simulink library "halin"  (R2021b)
settings: Solver=VariableStepAuto  StartTime=0.0  StopTime=10.0  RelTol=1e-3
undefined symbols (not defined in the file): TRUE
libraries: FVT_lib x177, hcu_lib x55
(part 12 of 17)

== system halin/HAL_IN/CAN5/VHAL_CANMsgInvalidTBOX1_flg ==
  Cast To Boolean13 : DataTypeConversion  OutDataTypeStr=boolean
  Constant : Constant  Value=TRUE
  Latch13 : hcu_lib/Basic_Blocks/Latch
  Switch13 : Switch  Criteria=u2 ~= 0
  Unit Delay : UnitDelay  SampleTime=-1  HasFrameUpgradeWarning=on
  UnitConverter : DataTypeConversion  OutDataTypeStr=boolean
  Out : Outport
  wires:
  Constant/1 -> Switch13/3
  Unit Delay/1 -> Cast To Boolean13/1
  Cast To Boolean13/1 -> Switch13/1, Latch13/1
  Switch13/1 -> UnitConverter/1
  Latch13/1 -> Switch13/2
  UnitConverter/1 -> Unit Delay/1, Out/1  "VHAL_CANMsgInvalidTBOX1_flg"

== system halin/HAL_IN/CAN5/VHAL_CANMsgInvalidTBOX2_flg ==
  Cast To Boolean13 : DataTypeConversion  OutDataTypeStr=boolean
  Constant : Constant  Value=TRUE
  Latch13 : hcu_lib/Basic_Blocks/Latch
  Switch13 : Switch  Criteria=u2 ~= 0
  Unit Delay : UnitDelay  SampleTime=-1  HasFrameUpgradeWarning=on
  UnitConverter : DataTypeConversion  OutDataTypeStr=boolean
  Out : Outport
  wires:
  Constant/1 -> Switch13/3
  Unit Delay/1 -> Cast To Boolean13/1
  Cast To Boolean13/1 -> Switch13/1, Latch13/1
  Switch13/1 -> UnitConverter/1
  Latch13/1 -> Switch13/2
  UnitConverter/1 -> Unit Delay/1, Out/1  "VHAL_CANMsgInvalidTBOX2_flg"

== system halin/HAL_IN/CAN5/VHAL_CANMsgInvalidTBOX3_flg ==
  Cast To Boolean13 : DataTypeConversion  OutDataTypeStr=boolean
  Constant : Constant  Value=TRUE
  Latch13 : hcu_lib/Basic_Blocks/Latch
  Switch13 : Switch  Criteria=u2 ~= 0
  Unit Delay : UnitDelay  SampleTime=-1  HasFrameUpgradeWarning=on
  UnitConverter : DataTypeConversion  OutDataTypeStr=boolean
  Out : Outport
  wires:
  Constant/1 -> Switch13/3
  Unit Delay/1 -> Cast To Boolean13/1
  Cast To Boolean13/1 -> Switch13/1, Latch13/1
  Switch13/1 -> UnitConverter/1
  Latch13/1 -> Switch13/2
  UnitConverter/1 -> Unit Delay/1, Out/1  "VHAL_CANMsgInvalidTBOX3_flg"

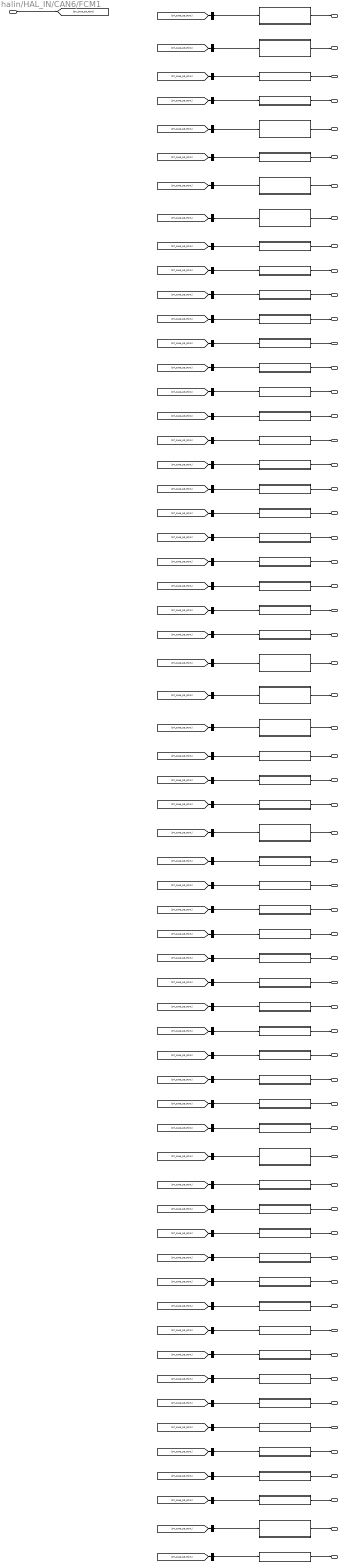
== system halin/HAL_IN/CAN6/FCM1 ==
  DT_CAN6_SG_FCM1 : Inport
  ACCComfortBandLower : Subsystem
  ACCComfortBandUpper : Subsystem
  ACCJerkLowerLimit : Subsystem
  ACCJerkUpperLimit : Subsystem
  ACCObjDist : Subsystem
  ACCObjDstLvl : Subsystem
  ACCObjRelSpd : Subsystem
  ACCRequiredAccel : Subsystem
  ACCTakeoverReq : Subsystem
  ACCVehHoldReq : Subsystem
  ADASACCSta : Subsystem
  ADASAEBReq : Subsystem
  ADASAEBSta : Subsystem
  ADASCAMSpdLim : Subsystem
  ADASDBSReq : Subsystem
  ADASFCWMute : Subsystem
  ADASFCWSta : Subsystem
  ADASFaultSta : Subsystem
  ADASFltWrnReq : Subsystem
  ADASForceIdle : Subsystem
  ADASISASta : Subsystem
  ADASLDWMute : Subsystem
  ADASLDWSta : Subsystem
  ADASLFCHandsOffWarning : Subsystem
  ADASLFCSta : Subsystem
  ADASLFCWarnSound : Subsystem
  ADASLKASta : Subsystem
  ADASLaneModeL : Subsystem
  ADASLaneModeR : Subsystem
  ADASLanecurveL : Subsystem
  ADASLanecurveR : Subsystem
  ADASLanetypeL : Subsystem
  ADASLanetypeR : Subsystem
  ADASSLIFSpdLim : Subsystem
  ADASSLIFSta : Subsystem
  ADASShftPosnReq : Subsystem
  ADASShftPosnReqA : Subsystem
  ADASVehSpdLim : Subsystem
  ADASWarningMsg : Subsystem
  AEBVehHoldReq : Subsystem
  CameraBlockage : Subsystem
  FCM1Checksum : Subsystem
  FCM1LifeCount : Subsystem
  FCMACCmode : Subsystem
  FCMLKAStrToqReq : Subsystem
  FCMLKATOIAct : Subsystem
  FCMLKATOIFault : Subsystem
  ForceLowBeam : Subsystem
  HazardWarningReq : Subsystem
  ISAWarningMsg : Subsystem
  LKAHODDisplayWarning : Subsystem
  LKAHODSoundWarning : Subsystem
  LVDAACCStatusInformation : Subsystem
  LVDADisabled : Subsystem
  LVDAFailinfo : Subsystem
  LVDAMuteSta : Subsystem
  LVDAWarning : Subsystem
  LeftTurnLightReq : Subsystem
  RightTurnLightReq : Subsystem
  TargetType : Subsystem
  TimeGapLevel : Subsystem
  bus_selector : BusSelector  OutputSignals=CAN6_ACC_ComfortBandLower
  bus_selector1 : BusSelector  OutputSignals=CAN6_ACC_ComfortBandUpper
  bus_selector10 : BusSelector  OutputSignals=CAN6_ADAS_ACC_Sta
  bus_selector11 : BusSelector  OutputSignals=CAN6_ADAS_AEBReq
  bus_selector12 : BusSelector  OutputSignals=CAN6_ADAS_AEB_Sta
  bus_selector13 : BusSelector  OutputSignals=CAN6_ADAS_CAM_SpdLim
  bus_selector14 : BusSelector  OutputSignals=CAN6_ADAS_DBSReq
  bus_selector15 : BusSelector  OutputSignals=CAN6_ADAS_FCW_Mute
  bus_selector16 : BusSelector  OutputSignals=CAN6_ADAS_FCW_Sta
  bus_selector17 : BusSelector  OutputSignals=CAN6_ADAS_FaultSta
  bus_selector18 : BusSelector  OutputSignals=CAN6_ADAS_FltWrnReq
  bus_selector19 : BusSelector  OutputSignals=CAN6_ADAS_ForceIdle
  bus_selector2 : BusSelector  OutputSignals=CAN6_ACC_JerkLowerLimit
  bus_selector20 : BusSelector  OutputSignals=CAN6_ADAS_ISA_Sta
  bus_selector21 : BusSelector  OutputSignals=CAN6_ADAS_LDW_Mute
  bus_selector22 : BusSelector  OutputSignals=CAN6_ADAS_LDW_Sta
  bus_selector23 : BusSelector  OutputSignals=CAN6_ADAS_LFC_Hands_Off_Warning
  bus_selector24 : BusSelector  OutputSignals=CAN6_ADAS_LFC_Sta
  bus_selector25 : BusSelector  OutputSignals=CAN6_ADAS_LFC_Warn_Sound
  bus_selector26 : BusSelector  OutputSignals=CAN6_ADAS_LKA_Sta
  bus_selector27 : BusSelector  OutputSignals=CAN6_ADAS_LaneModeL
  bus_selector28 : BusSelector  OutputSignals=CAN6_ADAS_LaneModeR
  bus_selector29 : BusSelector  OutputSignals=CAN6_ADAS_Lane_curveL
  bus_selector3 : BusSelector  OutputSignals=CAN6_ACC_JerkUpperLimit
  bus_selector30 : BusSelector  OutputSignals=CAN6_ADAS_Lane_curveR
  bus_selector31 : BusSelector  OutputSignals=CAN6_ADAS_LanetypeL
  bus_selector32 : BusSelector  OutputSignals=CAN6_ADAS_LanetypeR
  bus_selector33 : BusSelector  OutputSignals=CAN6_ADAS_SLIF_SpdLim
  bus_selector34 : BusSelector  OutputSignals=CAN6_ADAS_SLIF_Sta
  bus_selector35 : BusSelector  OutputSignals=CAN6_ADAS_ShftPosnReq
  bus_selector36 : BusSelector  OutputSignals=CAN6_ADAS_ShftPosnReq_A
  bus_selector37 : BusSelector  OutputSignals=CAN6_ADAS_VehSpdLim
  bus_selector38 : BusSelector  OutputSignals=CAN6_ADAS_WarningMsg
  bus_selector39 : BusSelector  OutputSignals=CAN6_AEB_VehHoldReq
  bus_selector4 : BusSelector  OutputSignals=CAN6_ACC_ObjDist
  bus_selector40 : BusSelector  OutputSignals=CAN6_CameraBlockage
  bus_selector41 : BusSelector  OutputSignals=CAN6_FCM1_Checksum
  bus_selector42 : BusSelector  OutputSignals=CAN6_FCM1_LifeCount
  bus_selector43 : BusSelector  OutputSignals=CAN6_FCM_ACCmode
  bus_selector44 : BusSelector  OutputSignals=CAN6_FCM_LKA_StrToqReq
  bus_selector45 : BusSelector  OutputSignals=CAN6_FCM_LKA_TOIAct
  bus_selector46 : BusSelector  OutputSignals=CAN6_FCM_LKA_TOIFault
  bus_selector47 : BusSelector  OutputSignals=CAN6_ForceLowBeam
  bus_selector48 : BusSelector  OutputSignals=CAN6_HazardWarningReq
  bus_selector49 : BusSelector  OutputSignals=CAN6_ISA_WarningMsg
  bus_selector5 : BusSelector  OutputSignals=CAN6_ACC_ObjDstLvl
  bus_selector50 : BusSelector  OutputSignals=CAN6_LKA_HOD_Display_Warning
  bus_selector51 : BusSelector  OutputSignals=CAN6_LKA_HOD_Sound_Warning
  bus_selector52 : BusSelector  OutputSignals=CAN6_LVDA_ACCStatusInformation
  bus_selector53 : BusSelector  OutputSignals=CAN6_LVDA_Disabled
  bus_selector54 : BusSelector  OutputSignals=CAN6_LVDA_Failinfo
  bus_selector55 : BusSelector  OutputSignals=CAN6_LVDA_Mute_Sta
  bus_selector56 : BusSelector  OutputSignals=CAN6_LVDA_Warning
  bus_selector57 : BusSelector  OutputSignals=CAN6_LeftTurnLightReq
  bus_selector58 : BusSelector  OutputSignals=CAN6_RightTurnLightReq
  bus_selector59 : BusSelector  OutputSignals=CAN6_Target_Type
  bus_selector6 : BusSelector  OutputSignals=CAN6_ACC_ObjRelSpd
  bus_selector60 : BusSelector  OutputSignals=CAN6_TimeGapLevel
  bus_selector7 : BusSelector  OutputSignals=CAN6_ACC_RequiredAccel
  bus_selector8 : BusSelector  OutputSignals=CAN6_ACC_TakeoverReq
  bus_selector9 : BusSelector  OutputSignals=CAN6_ACC_VehHoldReq
  VHAL_ACCComfortBandLower_mps2 : Outport
  VHAL_ACCComfortBandUpper_mps2 : Outport  Port=2
  VHAL_ACCJerkLowerLimit_mps3 : Outport  Port=3
  VHAL_ACCJerkUpperLimit_mps3 : Outport  Port=4
  VHAL_ACCObjDist_m : Outport  Port=5
  VHAL_ACCObjDstLvl_enum : Outport  Port=6
  VHAL_ACCObjRelSpd_mps : Outport  Port=7
  VHAL_ACCRequiredAccel_mps2 : Outport  Port=8
  VHAL_ACCTakeoverReq_flg : Outport  Port=9
  VHAL_ACCVehHoldReq_flg : Outport  Port=10
  VHAL_ADASACCSta_enum : Outport  Port=11
  VHAL_ADASAEBReq_enum : Outport  Port=12
  VHAL_ADASAEBSta_enum : Outport  Port=13
  VHAL_ADASCAMSpdLim_enum : Outport  Port=14
  VHAL_ADASDBSReq_enum : Outport  Port=15
  VHAL_ADASFCWMute_flg : Outport  Port=16
  VHAL_ADASFCWSta_enum : Outport  Port=17
  VHAL_ADASFaultSta_flg : Outport  Port=18
  VHAL_ADASFltWrnReq_flg : Outport  Port=19
  VHAL_ADASForceIdle_flg : Outport  Port=20
  VHAL_ADASISASta_enum : Outport  Port=21
  VHAL_ADASLDWMute_flg : Outport  Port=22
  VHAL_ADASLDWSta_enum : Outport  Port=23
  VHAL_ADASLFCHandsOffWarning_enum : Outport  Port=24
  VHAL_ADASLFCSta_enum : Outport  Port=25
  VHAL_ADASLFCWarnSound_enum : Outport  Port=26
  VHAL_ADASLKASta_enum : Outport  Port=27
  VHAL_ADASLaneModeL_enum : Outport  Port=28
  VHAL_ADASLaneModeR_enum : Outport  Port=29
  VHAL_ADASLanecurveL_raw32 : Outport  Port=30
  VHAL_ADASLanecurveR_raw32 : Outport  Port=31
  VHAL_ADASLanetypeL_enum : Outport  Port=32
  VHAL_ADASLanetypeR_enum : Outport  Port=33
  VHAL_ADASSLIFSpdLim_enum : Outport  Port=34
  VHAL_ADASSLIFSta_enum : Outport  Port=35
  VHAL_ADASShftPosnReq_enum : Outport  Port=36
  VHAL_ADASShftPosnReqA_flg : Outport  Port=37
  VHAL_ADASVehSpdLim_enum : Outport  Port=38
  VHAL_ADASWarningMsg_enum : Outport  Port=39
  VHAL_AEBVehHoldReq_flg : Outport  Port=40
  VHAL_CameraBlockage_flg : Outport  Port=41
  VHAL_FCM1Checksum_enum : Outport  Port=42
  VHAL_FCM1LifeCount_enum : Outport  Port=43
  VHAL_FCMACCmode_enum : Outport  Port=44
  VHAL_FCMLKAStrToqReq_Nm : Outport  Port=45
  VHAL_FCMLKATOIAct_enum : Outport  Port=46
  VHAL_FCMLKATOIFault_flg : Outport  Port=47
  VHAL_ForceLowBeam_enum : Outport  Port=48
  VHAL_HazardWarningReq_flg : Outport  Port=49
  VHAL_ISAWarningMsg_enum : Outport  Port=50
  VHAL_LKAHODDisplayWarning_flg : Outport  Port=51
  VHAL_LKAHODSoundWarning_flg : Outport  Port=52
  VHAL_LVDAACCStatusInformation_flg : Outport  Port=53
  VHAL_LVDADisabled_flg : Outport  Port=54
  VHAL_LVDAFailinfo_flg : Outport  Port=55
  VHAL_LVDAMuteSta_enum : Outport  Port=56
  VHAL_LVDAWarning_flg : Outport  Port=57
  VHAL_LeftTurnLightReq_flg : Outport  Port=58
  VHAL_RightTurnLightReq_flg : Outport  Port=59
  VHAL_TargetType_enum : Outport  Port=60
  VHAL_TimeGapLevel_enum : Outport  Port=61
  wires:
  DT_CAN6_SG_FCM1/1 -> [DT_CAN6_SG_FCM1]
  [DT_CAN6_SG_FCM1] -> bus_selector/1
  bus_selector/1 -> ACCComfortBandLower/1(ACC_ComfortBandLower)  "<CAN6_ACC_ComfortBandLower>"
  ACCComfortBandLower/1(VHAL_ACCComfortBandLower_mps2) -> VHAL_ACCComfortBandLower_mps2/1
  [DT_CAN6_SG_FCM1] -> bus_selector1/1
  bus_selector1/1 -> ACCComfortBandUpper/1(ACC_ComfortBandUpper)  "<CAN6_ACC_ComfortBandUpper>"
  ACCComfortBandUpper/1(VHAL_ACCComfortBandUpper_mps2) -> VHAL_ACCComfortBandUpper_mps2/1
  [DT_CAN6_SG_FCM1] -> bus_selector2/1
  bus_selector2/1 -> ACCJerkLowerLimit/1(ACC_JerkLowerLimit)  "<CAN6_ACC_JerkLowerLimit>"
  ACCJerkLowerLimit/1(VHAL_ACCJerkLowerLimit_mps3) -> VHAL_ACCJerkLowerLimit_mps3/1
  [DT_CAN6_SG_FCM1] -> bus_selector3/1
  bus_selector3/1 -> ACCJerkUpperLimit/1(ACC_JerkUpperLimit)  "<CAN6_ACC_JerkUpperLimit>"
  ACCJerkUpperLimit/1(VHAL_ACCJerkUpperLimit_mps3) -> VHAL_ACCJerkUpperLimit_mps3/1
  [DT_CAN6_SG_FCM1] -> bus_selector4/1
  bus_selector4/1 -> ACCObjDist/1(ACC_ObjDist)  "<CAN6_ACC_ObjDist>"
  ACCObjDist/1(VHAL_ACCObjDist_m) -> VHAL_ACCObjDist_m/1
  [DT_CAN6_SG_FCM1] -> bus_selector5/1
  bus_selector5/1 -> ACCObjDstLvl/1(ACC_ObjDstLvl)  "<CAN6_ACC_ObjDstLvl>"
  ACCObjDstLvl/1(VHAL_ACCObjDstLvl_enum) -> VHAL_ACCObjDstLvl_enum/1
  [DT_CAN6_SG_FCM1] -> bus_selector6/1
  bus_selector6/1 -> ACCObjRelSpd/1(ACC_ObjRelSpd)  "<CAN6_ACC_ObjRelSpd>"
  ACCObjRelSpd/1(VHAL_ACCObjRelSpd_mps) -> VHAL_ACCObjRelSpd_mps/1
  [DT_CAN6_SG_FCM1] -> bus_selector7/1
  bus_selector7/1 -> ACCRequiredAccel/1(ACC_RequiredAccel)  "<CAN6_ACC_RequiredAccel>"
  ACCRequiredAccel/1(VHAL_ACCRequiredAccel_mps2) -> VHAL_ACCRequiredAccel_mps2/1
  [DT_CAN6_SG_FCM1] -> bus_selector8/1
  bus_selector8/1 -> ACCTakeoverReq/1(ACC_TakeoverReq)  "<CAN6_ACC_TakeoverReq>"
  ACCTakeoverReq/1(VHAL_ACCTakeoverReq_flg) -> VHAL_ACCTakeoverReq_flg/1
  [DT_CAN6_SG_FCM1] -> bus_selector9/1
  bus_selector9/1 -> ACCVehHoldReq/1(ACC_VehHoldReq)  "<CAN6_ACC_VehHoldReq>"
  ACCVehHoldReq/1(VHAL_ACCVehHoldReq_flg) -> VHAL_ACCVehHoldReq_flg/1
  [DT_CAN6_SG_FCM1] -> bus_selector10/1
  bus_selector10/1 -> ADASACCSta/1(ADAS_ACC_Sta)  "<CAN6_ADAS_ACC_Sta>"
  ADASACCSta/1(VHAL_ADASACCSta_enum) -> VHAL_ADASACCSta_enum/1
  [DT_CAN6_SG_FCM1] -> bus_selector11/1
  bus_selector11/1 -> ADASAEBReq/1(ADAS_AEBReq)  "<CAN6_ADAS_AEBReq>"
  ADASAEBReq/1(VHAL_ADASAEBReq_enum) -> VHAL_ADASAEBReq_enum/1
  [DT_CAN6_SG_FCM1] -> bus_selector12/1
  bus_selector12/1 -> ADASAEBSta/1(ADAS_AEB_Sta)  "<CAN6_ADAS_AEB_Sta>"
  ADASAEBSta/1(VHAL_ADASAEBSta_enum) -> VHAL_ADASAEBSta_enum/1
  [DT_CAN6_SG_FCM1] -> bus_selector13/1
  bus_selector13/1 -> ADASCAMSpdLim/1(ADAS_CAM_SpdLim)  "<CAN6_ADAS_CAM_SpdLim>"
  ADASCAMSpdLim/1(VHAL_ADASCAMSpdLim_enum) -> VHAL_ADASCAMSpdLim_enum/1
  [DT_CAN6_SG_FCM1] -> bus_selector14/1
  bus_selector14/1 -> ADASDBSReq/1(ADAS_DBSReq)  "<CAN6_ADAS_DBSReq>"
  ADASDBSReq/1(VHAL_ADASDBSReq_enum) -> VHAL_ADASDBSReq_enum/1
  [DT_CAN6_SG_FCM1] -> bus_selector15/1
  bus_selector15/1 -> ADASFCWMute/1(ADAS_FCW_Mute)  "<CAN6_ADAS_FCW_Mute>"
  ADASFCWMute/1(VHAL_ADASFCWMute_flg) -> VHAL_ADASFCWMute_flg/1
  [DT_CAN6_SG_FCM1] -> bus_selector16/1
  bus_selector16/1 -> ADASFCWSta/1(ADAS_FCW_Sta)  "<CAN6_ADAS_FCW_Sta>"
  ADASFCWSta/1(VHAL_ADASFCWSta_enum) -> VHAL_ADASFCWSta_enum/1
  [DT_CAN6_SG_FCM1] -> bus_selector17/1
  bus_selector17/1 -> ADASFaultSta/1(ADAS_FaultSta)  "<CAN6_ADAS_FaultSta>"
  ADASFaultSta/1(VHAL_ADASFaultSta_flg) -> VHAL_ADASFaultSta_flg/1
  [DT_CAN6_SG_FCM1] -> bus_selector18/1
  bus_selector18/1 -> ADASFltWrnReq/1(ADAS_FltWrnReq)  "<CAN6_ADAS_FltWrnReq>"
  ADASFltWrnReq/1(VHAL_ADASFltWrnReq_flg) -> VHAL_ADASFltWrnReq_flg/1
  [DT_CAN6_SG_FCM1] -> bus_selector19/1
  bus_selector19/1 -> ADASForceIdle/1(ADAS_ForceIdle)  "<CAN6_ADAS_ForceIdle>"
  ADASForceIdle/1(VHAL_ADASForceIdle_flg) -> VHAL_ADASForceIdle_flg/1
  [DT_CAN6_SG_FCM1] -> bus_selector20/1
  bus_selector20/1 -> ADASISASta/1(ADAS_ISA_Sta)  "<CAN6_ADAS_ISA_Sta>"
  ADASISASta/1(VHAL_ADASISASta_enum) -> VHAL_ADASISASta_enum/1
  [DT_CAN6_SG_FCM1] -> bus_selector21/1
  bus_selector21/1 -> ADASLDWMute/1(ADAS_LDW_Mute)  "<CAN6_ADAS_LDW_Mute>"
  ADASLDWMute/1(VHAL_ADASLDWMute_flg) -> VHAL_ADASLDWMute_flg/1
  [DT_CAN6_SG_FCM1] -> bus_selector22/1
  bus_selector22/1 -> ADASLDWSta/1(ADAS_LDW_Sta)  "<CAN6_ADAS_LDW_Sta>"
  ADASLDWSta/1(VHAL_ADASLDWSta_enum) -> VHAL_ADASLDWSta_enum/1
  [DT_CAN6_SG_FCM1] -> bus_selector23/1
  bus_selector23/1 -> ADASLFCHandsOffWarning/1(ADAS_LFC_Hands_Off_Warning)  "<CAN6_ADAS_LFC_Hands_Off_Warning>"
  ADASLFCHandsOffWarning/1(VHAL_ADASLFCHandsOffWarning_enum) -> VHAL_ADASLFCHandsOffWarning_enum/1
  [DT_CAN6_SG_FCM1] -> bus_selector24/1
  bus_selector24/1 -> ADASLFCSta/1(ADAS_LFC_Sta)  "<CAN6_ADAS_LFC_Sta>"
  ADASLFCSta/1(VHAL_ADASLFCSta_enum) -> VHAL_ADASLFCSta_enum/1
  [DT_CAN6_SG_FCM1] -> bus_selector25/1
  bus_selector25/1 -> ADASLFCWarnSound/1(ADAS_LFC_Warn_Sound)  "<CAN6_ADAS_LFC_Warn_Sound>"
  ADASLFCWarnSound/1(VHAL_ADASLFCWarnSound_enum) -> VHAL_ADASLFCWarnSound_enum/1
  [DT_CAN6_SG_FCM1] -> bus_selector26/1
  bus_selector26/1 -> ADASLKASta/1(ADAS_LKA_Sta)  "<CAN6_ADAS_LKA_Sta>"
  ADASLKASta/1(VHAL_ADASLKASta_enum) -> VHAL_ADASLKASta_enum/1
  [DT_CAN6_SG_FCM1] -> bus_selector27/1
  bus_selector27/1 -> ADASLaneModeL/1(ADAS_LaneModeL)  "<CAN6_ADAS_LaneModeL>"
  ADASLaneModeL/1(VHAL_ADASLaneModeL_enum) -> VHAL_ADASLaneModeL_enum/1
  [DT_CAN6_SG_FCM1] -> bus_selector28/1
  bus_selector28/1 -> ADASLaneModeR/1(ADAS_LaneModeR)  "<CAN6_ADAS_LaneModeR>"
  ADASLaneModeR/1(VHAL_ADASLaneModeR_enum) -> VHAL_ADASLaneModeR_enum/1
  [DT_CAN6_SG_FCM1] -> bus_selector29/1
  bus_selector29/1 -> ADASLanecurveL/1(ADAS_Lane_curveL)  "<CAN6_ADAS_Lane_curveL>"
  ADASLanecurveL/1(VHAL_ADASLanecurveL_raw32) -> VHAL_ADASLanecurveL_raw32/1
  [DT_CAN6_SG_FCM1] -> bus_selector30/1
  bus_selector30/1 -> ADASLanecurveR/1(ADAS_Lane_curveR)  "<CAN6_ADAS_Lane_curveR>"
  ADASLanecurveR/1(VHAL_ADASLanecurveR_raw32) -> VHAL_ADASLanecurveR_raw32/1
  [DT_CAN6_SG_FCM1] -> bus_selector31/1
  bus_selector31/1 -> ADASLanetypeL/1(ADAS_LanetypeL)  "<CAN6_ADAS_LanetypeL>"
  ADASLanetypeL/1(VHAL_ADASLanetypeL_enum) -> VHAL_ADASLanetypeL_enum/1
  [DT_CAN6_SG_FCM1] -> bus_selector32/1
  bus_selector32/1 -> ADASLanetypeR/1(ADAS_LanetypeR)  "<CAN6_ADAS_LanetypeR>"
  ADASLanetypeR/1(VHAL_ADASLanetypeR_enum) -> VHAL_ADASLanetypeR_enum/1
  [DT_CAN6_SG_FCM1] -> bus_selector33/1
  bus_selector33/1 -> ADASSLIFSpdLim/1(ADAS_SLIF_SpdLim)  "<CAN6_ADAS_SLIF_SpdLim>"
  ADASSLIFSpdLim/1(VHAL_ADASSLIFSpdLim_enum) -> VHAL_ADASSLIFSpdLim_enum/1
  [DT_CAN6_SG_FCM1] -> bus_selector34/1
  bus_selector34/1 -> ADASSLIFSta/1(ADAS_SLIF_Sta)  "<CAN6_ADAS_SLIF_Sta>"
  ADASSLIFSta/1(VHAL_ADASSLIFSta_enum) -> VHAL_ADASSLIFSta_enum/1
  [DT_CAN6_SG_FCM1] -> bus_selector35/1
  bus_selector35/1 -> ADASShftPosnReq/1(ADAS_ShftPosnReq)  "<CAN6_ADAS_ShftPosnReq>"
  ADASShftPosnReq/1(VHAL_ADASShftPosnReq_enum) -> VHAL_ADASShftPosnReq_enum/1
  [DT_CAN6_SG_FCM1] -> bus_selector36/1
  bus_selector36/1 -> ADASShftPosnReqA/1(ADAS_ShftPosnReq_A)  "<CAN6_ADAS_ShftPosnReq_A>"
  ADASShftPosnReqA/1(VHAL_ADASShftPosnReqA_flg) -> VHAL_ADASShftPosnReqA_flg/1
  [DT_CAN6_SG_FCM1] -> bus_selector37/1
  bus_selector37/1 -> ADASVehSpdLim/1(ADAS_VehSpdLim)  "<CAN6_ADAS_VehSpdLim>"
  ADASVehSpdLim/1(VHAL_ADASVehSpdLim_enum) -> VHAL_ADASVehSpdLim_enum/1
  [DT_CAN6_SG_FCM1] -> bus_selector38/1
  bus_selector38/1 -> ADASWarningMsg/1(ADAS_WarningMsg)  "<CAN6_ADAS_WarningMsg>"
  ADASWarningMsg/1(VHAL_ADASWarningMsg_enum) -> VHAL_ADASWarningMsg_enum/1
  [DT_CAN6_SG_FCM1] -> bus_selector39/1
  bus_selector39/1 -> AEBVehHoldReq/1(AEB_VehHoldReq)  "<CAN6_AEB_VehHoldReq>"
  AEBVehHoldReq/1(VHAL_AEBVehHoldReq_flg) -> VHAL_AEBVehHoldReq_flg/1
  [DT_CAN6_SG_FCM1] -> bus_selector40/1
  bus_selector40/1 -> CameraBlockage/1(CameraBlockage)  "<CAN6_CameraBlockage>"
  CameraBlockage/1(VHAL_CameraBlockage_flg) -> VHAL_CameraBlockage_flg/1
  [DT_CAN6_SG_FCM1] -> bus_selector41/1
  bus_selector41/1 -> FCM1Checksum/1(FCM1_Checksum)  "<CAN6_FCM1_Checksum>"
  FCM1Checksum/1(VHAL_FCM1Checksum_enum) -> VHAL_FCM1Checksum_enum/1
  [DT_CAN6_SG_FCM1] -> bus_selector42/1
  bus_selector42/1 -> FCM1LifeCount/1(FCM1_LifeCount)  "<CAN6_FCM1_LifeCount>"
  FCM1LifeCount/1(VHAL_FCM1LifeCount_enum) -> VHAL_FCM1LifeCount_enum/1
  [DT_CAN6_SG_FCM1] -> bus_selector43/1
  bus_selector43/1 -> FCMACCmode/1(FCM_ACCmode)  "<CAN6_FCM_ACCmode>"
  FCMACCmode/1(VHAL_FCMACCmode_enum) -> VHAL_FCMACCmode_enum/1
  [DT_CAN6_SG_FCM1] -> bus_selector44/1
  bus_selector44/1 -> FCMLKAStrToqReq/1(FCM_LKA_StrToqReq)  "<CAN6_FCM_LKA_StrToqReq>"
  FCMLKAStrToqReq/1(VHAL_FCMLKAStrToqReq_Nm) -> VHAL_FCMLKAStrToqReq_Nm/1
  [DT_CAN6_SG_FCM1] -> bus_selector45/1
  bus_selector45/1 -> FCMLKATOIAct/1(FCM_LKA_TOIAct)  "<CAN6_FCM_LKA_TOIAct>"
  FCMLKATOIAct/1(VHAL_FCMLKATOIAct_enum) -> VHAL_FCMLKATOIAct_enum/1
  [DT_CAN6_SG_FCM1] -> bus_selector46/1
  bus_selector46/1 -> FCMLKATOIFault/1(FCM_LKA_TOIFault)  "<CAN6_FCM_LKA_TOIFault>"
  FCMLKATOIFault/1(VHAL_FCMLKATOIFault_flg) -> VHAL_FCMLKATOIFault_flg/1
  [DT_CAN6_SG_FCM1] -> bus_selector47/1
  bus_selector47/1 -> ForceLowBeam/1(ForceLowBeam)  "<CAN6_ForceLowBeam>"
  ForceLowBeam/1(VHAL_ForceLowBeam_enum) -> VHAL_ForceLowBeam_enum/1
  [DT_CAN6_SG_FCM1] -> bus_selector48/1
  bus_selector48/1 -> HazardWarningReq/1(HazardWarningReq)  "<CAN6_HazardWarningReq>"
  HazardWarningReq/1(VHAL_HazardWarningReq_flg) -> VHAL_HazardWarningReq_flg/1
  [DT_CAN6_SG_FCM1] -> bus_selector49/1
  bus_selector49/1 -> ISAWarningMsg/1(ISA_WarningMsg)  "<CAN6_ISA_WarningMsg>"
  ISAWarningMsg/1(VHAL_ISAWarningMsg_enum) -> VHAL_ISAWarningMsg_enum/1
  [DT_CAN6_SG_FCM1] -> bus_selector50/1
  bus_selector50/1 -> LKAHODDisplayWarning/1(LKA_HOD_Display_Warning)  "<CAN6_LKA_HOD_Display_Warning>"
  LKAHODDisplayWarning/1(VHAL_LKAHODDisplayWarning_flg) -> VHAL_LKAHODDisplayWarning_flg/1
  [DT_CAN6_SG_FCM1] -> bus_selector51/1
  bus_selector51/1 -> LKAHODSoundWarning/1(LKA_HOD_Sound_Warning)  "<CAN6_LKA_HOD_Sound_Warning>"
  LKAHODSoundWarning/1(VHAL_LKAHODSoundWarning_flg) -> VHAL_LKAHODSoundWarning_flg/1
  [DT_CAN6_SG_FCM1] -> bus_selector52/1
  bus_selector52/1 -> LVDAACCStatusInformation/1(LVDA_ACCStatusInformation)  "<CAN6_LVDA_ACCStatusInformation>"
  LVDAACCStatusInformation/1(VHAL_LVDAACCStatusInformation_flg) -> VHAL_LVDAACCStatusInformation_flg/1
  [DT_CAN6_SG_FCM1] -> bus_selector53/1
  bus_selector53/1 -> LVDADisabled/1(LVDA_Disabled)  "<CAN6_LVDA_Disabled>"
  LVDADisabled/1(VHAL_LVDADisabled_flg) -> VHAL_LVDADisabled_flg/1
  [DT_CAN6_SG_FCM1] -> bus_selector54/1
  bus_selector54/1 -> LVDAFailinfo/1(LVDA_Failinfo)  "<CAN6_LVDA_Failinfo>"
  LVDAFailinfo/1(VHAL_LVDAFailinfo_flg) -> VHAL_LVDAFailinfo_flg/1
  [DT_CAN6_SG_FCM1] -> bus_selector55/1
  bus_selector55/1 -> LVDAMuteSta/1(LVDA_Mute_Sta)  "<CAN6_LVDA_Mute_Sta>"
  LVDAMuteSta/1(VHAL_LVDAMuteSta_enum) -> VHAL_LVDAMuteSta_enum/1
  [DT_CAN6_SG_FCM1] -> bus_selector56/1
  bus_selector56/1 -> LVDAWarning/1(LVDA_Warning)  "<CAN6_LVDA_Warning>"
  LVDAWarning/1(VHAL_LVDAWarning_flg) -> VHAL_LVDAWarning_flg/1
  [DT_CAN6_SG_FCM1] -> bus_selector57/1
  bus_selector57/1 -> LeftTurnLightReq/1(LeftTurnLightReq)  "<CAN6_LeftTurnLightReq>"
  LeftTurnLightReq/1(VHAL_LeftTurnLightReq_flg) -> VHAL_LeftTurnLightReq_flg/1
  [DT_CAN6_SG_FCM1] -> bus_selector58/1
  bus_selector58/1 -> RightTurnLightReq/1(RightTurnLightReq)  "<CAN6_RightTurnLightReq>"
  RightTurnLightReq/1(VHAL_RightTurnLightReq_flg) -> VHAL_RightTurnLightReq_flg/1
  [DT_CAN6_SG_FCM1] -> bus_selector59/1
  bus_selector59/1 -> TargetType/1(Target_Type)  "<CAN6_Target_Type>"
  TargetType/1(VHAL_TargetType_enum) -> VHAL_TargetType_enum/1
  [DT_CAN6_SG_FCM1] -> bus_selector60/1
  bus_selector60/1 -> TimeGapLevel/1(TimeGapLevel)  "<CAN6_TimeGapLevel>"
  TimeGapLevel/1(VHAL_TimeGapLevel_enum) -> VHAL_TimeGapLevel_enum/1

== system halin/HAL_IN/CAN6/FCM3 ==
  DT_CAN6_SG_FCM3 : Inport
  MELaneCurvDervLt : Subsystem
  MELaneCurvDervLt2 : Subsystem
  MELaneCurvDervRt : Subsystem
  MELaneCurvDervRt2 : Subsystem
  MELaneCurvLt : Subsystem
  MELaneCurvLt2 : Subsystem
  MELaneCurvRt : Subsystem
  MELaneCurvRt2 : Subsystem
  MELaneHeadAngLt : Subsystem
  MELaneHeadAngLt2 : Subsystem
  MELaneHeadAngRt : Subsystem
  MELaneHeadAngRt2 : Subsystem
  MELanePosLt : Subsystem
  MELanePosLt2 : Subsystem
  MELanePosRt : Subsystem
  MELanePosRt2 : Subsystem
  bus_selector : BusSelector  OutputSignals=CAN6_ME_Lane_CurvDervLt
  bus_selector1 : BusSelector  OutputSignals=CAN6_ME_Lane_CurvDervLt2
  bus_selector10 : BusSelector  OutputSignals=CAN6_ME_Lane_HeadAngRt
  bus_selector11 : BusSelector  OutputSignals=CAN6_ME_Lane_HeadAngRt2
  bus_selector12 : BusSelector  OutputSignals=CAN6_ME_Lane_PosLt
  bus_selector13 : BusSelector  OutputSignals=CAN6_ME_Lane_PosLt2
  bus_selector14 : BusSelector  OutputSignals=CAN6_ME_Lane_PosRt
  bus_selector15 : BusSelector  OutputSignals=CAN6_ME_Lane_PosRt2
  bus_selector2 : BusSelector  OutputSignals=CAN6_ME_Lane_CurvDervRt
  bus_selector3 : BusSelector  OutputSignals=CAN6_ME_Lane_CurvDervRt2
  bus_selector4 : BusSelector  OutputSignals=CAN6_ME_Lane_CurvLt
  bus_selector5 : BusSelector  OutputSignals=CAN6_ME_Lane_CurvLt2
  bus_selector6 : BusSelector  OutputSignals=CAN6_ME_Lane_CurvRt
  bus_selector7 : BusSelector  OutputSignals=CAN6_ME_Lane_CurvRt2
  bus_selector8 : BusSelector  OutputSignals=CAN6_ME_Lane_HeadAngLt
  bus_selector9 : BusSelector  OutputSignals=CAN6_ME_Lane_HeadAngLt2
  VHAL_MELaneCurvDervLt_raw32 : Outport
  VHAL_MELaneCurvDervLt2_raw32 : Outport  Port=2
  VHAL_MELaneCurvDervRt_raw32 : Outport  Port=3
  VHAL_MELaneCurvDervRt2_raw32 : Outport  Port=4
  VHAL_MELaneCurvLt_raw32 : Outport  Port=5
  VHAL_MELaneCurvLt2_raw32 : Outport  Port=6
  VHAL_MELaneCurvRt_raw32 : Outport  Port=7
  VHAL_MELaneCurvRt2_raw32 : Outport  Port=8
  VHAL_MELaneHeadAngLt_radians : Outport  Port=9
  VHAL_MELaneHeadAngLt2_radians : Outport  Port=10
  VHAL_MELaneHeadAngRt_radians : Outport  Port=11
  VHAL_MELaneHeadAngRt2_radians : Outport  Port=12
  VHAL_MELanePosLt_m : Outport  Port=13
  VHAL_MELanePosLt2_m : Outport  Port=14
  VHAL_MELanePosRt_m : Outport  Port=15
  VHAL_MELanePosRt2_m : Outport  Port=16
  wires:
  DT_CAN6_SG_FCM3/1 -> [DT_CAN6_SG_FCM3]
  [DT_CAN6_SG_FCM3] -> bus_selector/1
  bus_selector/1 -> MELaneCurvDervLt/1(ME_Lane_CurvDervLt)  "<CAN6_ME_Lane_CurvDervLt>"
  MELaneCurvDervLt/1(VHAL_MELaneCurvDervLt_raw32) -> VHAL_MELaneCurvDervLt_raw32/1
  [DT_CAN6_SG_FCM3] -> bus_selector1/1
  bus_selector1/1 -> MELaneCurvDervLt2/1(ME_Lane_CurvDervLt2)  "<CAN6_ME_Lane_CurvDervLt2>"
  MELaneCurvDervLt2/1(VHAL_MELaneCurvDervLt2_raw32) -> VHAL_MELaneCurvDervLt2_raw32/1
  [DT_CAN6_SG_FCM3] -> bus_selector2/1
  bus_selector2/1 -> MELaneCurvDervRt/1(ME_Lane_CurvDervRt)  "<CAN6_ME_Lane_CurvDervRt>"
  MELaneCurvDervRt/1(VHAL_MELaneCurvDervRt_raw32) -> VHAL_MELaneCurvDervRt_raw32/1
  [DT_CAN6_SG_FCM3] -> bus_selector3/1
  bus_selector3/1 -> MELaneCurvDervRt2/1(ME_Lane_CurvDervRt2)  "<CAN6_ME_Lane_CurvDervRt2>"
  MELaneCurvDervRt2/1(VHAL_MELaneCurvDervRt2_raw32) -> VHAL_MELaneCurvDervRt2_raw32/1
  [DT_CAN6_SG_FCM3] -> bus_selector4/1
  bus_selector4/1 -> MELaneCurvLt/1(ME_Lane_CurvLt)  "<CAN6_ME_Lane_CurvLt>"
  MELaneCurvLt/1(VHAL_MELaneCurvLt_raw32) -> VHAL_MELaneCurvLt_raw32/1
  [DT_CAN6_SG_FCM3] -> bus_selector5/1
  bus_selector5/1 -> MELaneCurvLt2/1(ME_Lane_CurvLt2)  "<CAN6_ME_Lane_CurvLt2>"
  MELaneCurvLt2/1(VHAL_MELaneCurvLt2_raw32) -> VHAL_MELaneCurvLt2_raw32/1
  [DT_CAN6_SG_FCM3] -> bus_selector6/1
  bus_selector6/1 -> MELaneCurvRt/1(ME_Lane_CurvRt)  "<CAN6_ME_Lane_CurvRt>"
  MELaneCurvRt/1(VHAL_MELaneCurvRt_raw32) -> VHAL_MELaneCurvRt_raw32/1
  [DT_CAN6_SG_FCM3] -> bus_selector7/1
  bus_selector7/1 -> MELaneCurvRt2/1(ME_Lane_CurvRt2)  "<CAN6_ME_Lane_CurvRt2>"
  MELaneCurvRt2/1(VHAL_MELaneCurvRt2_raw32) -> VHAL_MELaneCurvRt2_raw32/1
  [DT_CAN6_SG_FCM3] -> bus_selector8/1
  bus_selector8/1 -> MELaneHeadAngLt/1(ME_Lane_HeadAngLt)  "<CAN6_ME_Lane_HeadAngLt>"
  MELaneHeadAngLt/1(VHAL_MELaneHeadAngLt_radians) -> VHAL_MELaneHeadAngLt_radians/1
  [DT_CAN6_SG_FCM3] -> bus_selector9/1
  bus_selector9/1 -> MELaneHeadAngLt2/1(ME_Lane_HeadAngLt2)  "<CAN6_ME_Lane_HeadAngLt2>"
  MELaneHeadAngLt2/1(VHAL_MELaneHeadAngLt2_radians) -> VHAL_MELaneHeadAngLt2_radians/1
  [DT_CAN6_SG_FCM3] -> bus_selector10/1
  bus_selector10/1 -> MELaneHeadAngRt/1(ME_Lane_HeadAngRt)  "<CAN6_ME_Lane_HeadAngRt>"
  MELaneHeadAngRt/1(VHAL_MELaneHeadAngRt_radians) -> VHAL_MELaneHeadAngRt_radians/1
  [DT_CAN6_SG_FCM3] -> bus_selector11/1
  bus_selector11/1 -> MELaneHeadAngRt2/1(ME_Lane_HeadAngRt2)  "<CAN6_ME_Lane_HeadAngRt2>"
  MELaneHeadAngRt2/1(VHAL_MELaneHeadAngRt2_radians) -> VHAL_MELaneHeadAngRt2_radians/1
  [DT_CAN6_SG_FCM3] -> bus_selector12/1
  bus_selector12/1 -> MELanePosLt/1(ME_Lane_PosLt)  "<CAN6_ME_Lane_PosLt>"
  MELanePosLt/1(VHAL_MELanePosLt_m) -> VHAL_MELanePosLt_m/1
  [DT_CAN6_SG_FCM3] -> bus_selector13/1
  bus_selector13/1 -> MELanePosLt2/1(ME_Lane_PosLt2)  "<CAN6_ME_Lane_PosLt2>"
  MELanePosLt2/1(VHAL_MELanePosLt2_m) -> VHAL_MELanePosLt2_m/1
  [DT_CAN6_SG_FCM3] -> bus_selector14/1
  bus_selector14/1 -> MELanePosRt/1(ME_Lane_PosRt)  "<CAN6_ME_Lane_PosRt>"
  MELanePosRt/1(VHAL_MELanePosRt_m) -> VHAL_MELanePosRt_m/1
  [DT_CAN6_SG_FCM3] -> bus_selector15/1
  bus_selector15/1 -> MELanePosRt2/1(ME_Lane_PosRt2)  "<CAN6_ME_Lane_PosRt2>"
  MELanePosRt2/1(VHAL_MELanePosRt2_m) -> VHAL_MELanePosRt2_m/1

== system halin/HAL_IN/CAN6/SRR1 ==
  DT_CAN6_SG_SRR1 : Inport
  SRRBSDWarnL : Subsystem
  SRRBSDWarnR : Subsystem
  SRRODAWarnL : Subsystem
  SRRODAWarnR : Subsystem
  bus_selector : BusSelector  OutputSignals=CAN6_SRR_BSD_WarnL
  bus_selector1 : BusSelector  OutputSignals=CAN6_SRR_BSD_WarnR
  bus_selector2 : BusSelector  OutputSignals=CAN6_SRR_ODA_WarnL
  bus_selector3 : BusSelector  OutputSignals=CAN6_SRR_ODA_WarnR
  VHAL_SRRBSDWarnL_enum : Outport
  VHAL_SRRBSDWarnR_enum : Outport  Port=2
  VHAL_SRRODAWarnL_enum : Outport  Port=3
  VHAL_SRRODAWarnR_enum : Outport  Port=4
  wires:
  DT_CAN6_SG_SRR1/1 -> [DT_CAN6_SG_SRR1]
  [DT_CAN6_SG_SRR1] -> bus_selector/1
  bus_selector/1 -> SRRBSDWarnL/1(SRR_BSD_WarnL)  "<CAN6_SRR_BSD_WarnL>"
  SRRBSDWarnL/1(VHAL_SRRBSDWarnL_enum) -> VHAL_SRRBSDWarnL_enum/1
  [DT_CAN6_SG_SRR1] -> bus_selector1/1
  bus_selector1/1 -> SRRBSDWarnR/1(SRR_BSD_WarnR)  "<CAN6_SRR_BSD_WarnR>"
  SRRBSDWarnR/1(VHAL_SRRBSDWarnR_enum) -> VHAL_SRRBSDWarnR_enum/1
  [DT_CAN6_SG_SRR1] -> bus_selector2/1
  bus_selector2/1 -> SRRODAWarnL/1(SRR_ODA_WarnL)  "<CAN6_SRR_ODA_WarnL>"
  SRRODAWarnL/1(VHAL_SRRODAWarnL_enum) -> VHAL_SRRODAWarnL_enum/1
  [DT_CAN6_SG_SRR1] -> bus_selector3/1
  bus_selector3/1 -> SRRODAWarnR/1(SRR_ODA_WarnR)  "<CAN6_SRR_ODA_WarnR>"
  SRRODAWarnR/1(VHAL_SRRODAWarnR_enum) -> VHAL_SRRODAWarnR_enum/1

== system halin/HAL_IN/CAN6/VHAL_CANMsgInvalidFCM1_flg ==
  Cast To Boolean13 : DataTypeConversion  OutDataTypeStr=boolean
  Constant : Constant  Value=TRUE
  Latch13 : hcu_lib/Basic_Blocks/Latch
  Switch13 : Switch  Criteria=u2 ~= 0
  Unit Delay : UnitDelay  SampleTime=-1  HasFrameUpgradeWarning=on
  UnitConverter : DataTypeConversion  OutDataTypeStr=boolean
  Out : Outport
  wires:
  Constant/1 -> Switch13/3
  Unit Delay/1 -> Cast To Boolean13/1
  Cast To Boolean13/1 -> Switch13/1, Latch13/1
  Switch13/1 -> UnitConverter/1
  Latch13/1 -> Switch13/2
  UnitConverter/1 -> Unit Delay/1, Out/1  "VHAL_CANMsgInvalidFCM1_flg"

== system halin/HAL_IN/CAN6/VHAL_CANMsgInvalidFCM3_flg ==
  Cast To Boolean13 : DataTypeConversion  OutDataTypeStr=boolean
  Constant : Constant  Value=TRUE
  Latch13 : hcu_lib/Basic_Blocks/Latch
  Switch13 : Switch  Criteria=u2 ~= 0
  Unit Delay : UnitDelay  SampleTime=-1  HasFrameUpgradeWarning=on
  UnitConverter : DataTypeConversion  OutDataTypeStr=boolean
  Out : Outport
  wires:
  Constant/1 -> Switch13/3
  Unit Delay/1 -> Cast To Boolean13/1
  Cast To Boolean13/1 -> Switch13/1, Latch13/1
  Switch13/1 -> UnitConverter/1
  Latch13/1 -> Switch13/2
  UnitConverter/1 -> Unit Delay/1, Out/1  "VHAL_CANMsgInvalidFCM3_flg"

== system halin/HAL_IN/CAN6/VHAL_CANMsgInvalidSRR1_flg ==
  Cast To Boolean13 : DataTypeConversion  OutDataTypeStr=boolean
  Constant : Constant  Value=TRUE
  Latch13 : hcu_lib/Basic_Blocks/Latch
  Switch13 : Switch  Criteria=u2 ~= 0
  Unit Delay : UnitDelay  SampleTime=-1  HasFrameUpgradeWarning=on
  UnitConverter : DataTypeConversion  OutDataTypeStr=boolean
  Out : Outport
  wires:
  Constant/1 -> Switch13/3
  Unit Delay/1 -> Cast To Boolean13/1
  Cast To Boolean13/1 -> Switch13/1, Latch13/1
  Switch13/1 -> UnitConverter/1
  Latch13/1 -> Switch13/2
  UnitConverter/1 -> Unit Delay/1, Out/1  "VHAL_CANMsgInvalidSRR1_flg"

== system halin/HAL_IN/CAN1/ABM1/ABMPassengerODSSta ==
  ABM_Passenger_ODS_Sta : Inport
  UnitConverter : DataTypeConversion  OutDataTypeStr=uint8
  VHAL_ABMPassengerODSSta_flg : Outport
  wires:
  UnitConverter/1 -> VHAL_ABMPassengerODSSta_flg/1
  ABM_Passenger_ODS_Sta/1 -> UnitConverter/1

== system halin/HAL_IN/CAN1/ABM1/ABMRearPassengerCTRODSSta ==
  ABM_RearPassengerCTR_ODS_Sta : Inport
  UnitConverter : DataTypeConversion  OutDataTypeStr=uint8
  VHAL_ABMRearPassengerCTRODSSta_flg : Outport
  wires:
  UnitConverter/1 -> VHAL_ABMRearPassengerCTRODSSta_flg/1
  ABM_RearPassengerCTR_ODS_Sta/1 -> UnitConverter/1

== system halin/HAL_IN/CAN1/ABM1/ABMRearPassengerLHODSSta ==
  ABM_RearPassengerLH_ODS_Sta : Inport
  UnitConverter : DataTypeConversion  OutDataTypeStr=uint8
  VHAL_ABMRearPassengerLHODSSta_flg : Outport
  wires:
  UnitConverter/1 -> VHAL_ABMRearPassengerLHODSSta_flg/1
  ABM_RearPassengerLH_ODS_Sta/1 -> UnitConverter/1

== system halin/HAL_IN/CAN1/ABM1/ABMRearPassengerRHODSSta ==
  ABM_RearPassengerRH_ODS_Sta : Inport
  UnitConverter : DataTypeConversion  OutDataTypeStr=uint8
  VHAL_ABMRearPassengerRHODSSta_flg : Outport
  wires:
  UnitConverter/1 -> VHAL_ABMRearPassengerRHODSSta_flg/1
  ABM_RearPassengerRH_ODS_Sta/1 -> UnitConverter/1

== system halin/HAL_IN/CAN1/ABM1/AirBagFailCmd ==
  AirBagFailCmd : Inport
  UnitConverter : DataTypeConversion  OutDataTypeStr=uint8
  VHAL_AirBagFailCmd_flg : Outport
  wires:
  UnitConverter/1 -> VHAL_AirBagFailCmd_flg/1
  AirBagFailCmd/1 -> UnitConverter/1

== system halin/HAL_IN/CAN1/ABM1/ChecksumABM1 ==
  Checksum_ABM1 : Inport
  UnitConverter : DataTypeConversion  OutDataTypeStr=uint8
  VHAL_ChecksumABM1_enum : Outport
  wires:
  UnitConverter/1 -> VHAL_ChecksumABM1_enum/1
  Checksum_ABM1/1 -> UnitConverter/1

== system halin/HAL_IN/CAN1/ABM1/CrashOutputSts ==
  CrashOutputSts : Inport
  UnitConverter : DataTypeConversion  OutDataTypeStr=uint8
  VHAL_CrashOutputSts_enum : Outport
  wires:
  UnitConverter/1 -> VHAL_CrashOutputSts_enum/1
  CrashOutputSts/1 -> UnitConverter/1

== system halin/HAL_IN/CAN1/ABM1/DriverSeatBeltCmd ==
  DriverSeatBeltCmd : Inport
  UnitConverter : DataTypeConversion  OutDataTypeStr=uint8
  VHAL_DriverSeatBeltCmd_flg : Outport
  wires:
  UnitConverter/1 -> VHAL_DriverSeatBeltCmd_flg/1
  DriverSeatBeltCmd/1 -> UnitConverter/1

== system halin/HAL_IN/CAN1/ABM1/LifeCountABM1 ==
  LifeCount_ABM1 : Inport
  UnitConverter : DataTypeConversion  OutDataTypeStr=uint8
  VHAL_LifeCountABM1_enum : Outport
  wires:
  UnitConverter/1 -> VHAL_LifeCountABM1_enum/1
  LifeCount_ABM1/1 -> UnitConverter/1

== system halin/HAL_IN/CAN1/ABM1/PABSwitchCmd ==
  PABSwitchCmd : Inport
  UnitConverter : DataTypeConversion  OutDataTypeStr=uint8
  VHAL_PABSwitchCmd_flg : Outport
  wires:
  UnitConverter/1 -> VHAL_PABSwitchCmd_flg/1
  PABSwitchCmd/1 -> UnitConverter/1

== system halin/HAL_IN/CAN1/ABM1/PsngrSeatBeltCmd ==
  PsngrSeatBeltCmd : Inport
  UnitConverter : DataTypeConversion  OutDataTypeStr=uint8
  VHAL_PsngrSeatBeltCmd_flg : Outport
  wires:
  UnitConverter/1 -> VHAL_PsngrSeatBeltCmd_flg/1
  PsngrSeatBeltCmd/1 -> UnitConverter/1

== system halin/HAL_IN/CAN1/ABM1/RCenterSeatBeltCmd ==
  RCenterSeatBeltCmd : Inport
  UnitConverter : DataTypeConversion  OutDataTypeStr=uint8
  VHAL_RCenterSeatBeltCmd_flg : Outport
  wires:
  UnitConverter/1 -> VHAL_RCenterSeatBeltCmd_flg/1
  RCenterSeatBeltCmd/1 -> UnitConverter/1

== system halin/HAL_IN/CAN1/ABM1/RDriverSeatBeltCmd ==
  RDriverSeatBeltCmd : Inport
  UnitConverter : DataTypeConversion  OutDataTypeStr=uint8
  VHAL_RDriverSeatBeltCmd_flg : Outport
  wires:
  UnitConverter/1 -> VHAL_RDriverSeatBeltCmd_flg/1
  RDriverSeatBeltCmd/1 -> UnitConverter/1

== system halin/HAL_IN/CAN1/ABM1/RPsngrSeatBeltCmd ==
  RPsngrSeatBeltCmd : Inport
  UnitConverter : DataTypeConversion  OutDataTypeStr=uint8
  VHAL_RPsngrSeatBeltCmd_flg : Outport
  wires:
  UnitConverter/1 -> VHAL_RPsngrSeatBeltCmd_flg/1
  RPsngrSeatBeltCmd/1 -> UnitConverter/1

== system halin/HAL_IN/CAN1/ABM1/TLHPsngrSeatBeltCmd ==
  TLHPsngrSeatBeltCmd : Inport
  UnitConverter : DataTypeConversion  OutDataTypeStr=uint8
  VHAL_TLHPsngrSeatBeltCmd_flg : Outport
  wires:
  UnitConverter/1 -> VHAL_TLHPsngrSeatBeltCmd_flg/1
  TLHPsngrSeatBeltCmd/1 -> UnitConverter/1

== system halin/HAL_IN/CAN1/ABM1/TRHPsngrSeatBeltCmd ==
  TRHPsngrSeatBeltCmd : Inport
  UnitConverter : DataTypeConversion  OutDataTypeStr=uint8
  VHAL_TRHPsngrSeatBeltCmd_flg : Outport
  wires:
  UnitConverter/1 -> VHAL_TRHPsngrSeatBeltCmd_flg/1
  TRHPsngrSeatBeltCmd/1 -> UnitConverter/1

== system halin/HAL_IN/CAN1/EPB1/DOASta ==
  DOA_Sta : Inport
  UnitConverter : DataTypeConversion  OutDataTypeStr=uint8
  VHAL_DOASta_flg : Outport
  wires:
  UnitConverter/1 -> VHAL_DOASta_flg/1
  DOA_Sta/1 -> UnitConverter/1

== system halin/HAL_IN/CAN1/EPB1/EPBCarWashMode ==
  EPBCarWashMode : Inport
  UnitConverter : DataTypeConversion  OutDataTypeStr=uint8
  VHAL_EPBCarWashMode_flg : Outport
  wires:
  UnitConverter/1 -> VHAL_EPBCarWashMode_flg/1
  EPBCarWashMode/1 -> UnitConverter/1

== system halin/HAL_IN/CAN1/EPB1/EPBErrSta ==
  EPBErrSta : Inport
  UnitConverter : DataTypeConversion  OutDataTypeStr=uint8
  VHAL_EPBErrSta_enum : Outport
  wires:
  UnitConverter/1 -> VHAL_EPBErrSta_enum/1
  EPBErrSta/1 -> UnitConverter/1

== system halin/HAL_IN/CAN1/EPB1/EPBExtApplyAvail ==
  EPBExtApplyAvail : Inport
  UnitConverter : DataTypeConversion  OutDataTypeStr=uint8
  VHAL_EPBExtApplyAvail_flg : Outport
  wires:
  UnitConverter/1 -> VHAL_EPBExtApplyAvail_flg/1
  EPBExtApplyAvail/1 -> UnitConverter/1

== system halin/HAL_IN/CAN1/EPB1/EPBExtReleaseAvail ==
  EPBExtReleaseAvail : Inport
  UnitConverter : DataTypeConversion  OutDataTypeStr=uint8
  VHAL_EPBExtReleaseAvail_flg : Outport
  wires:
  UnitConverter/1 -> VHAL_EPBExtReleaseAvail_flg/1
  EPBExtReleaseAvail/1 -> UnitConverter/1

== system halin/HAL_IN/CAN1/EPB1/EPBSta ==
  EPBSta : Inport
  UnitConverter : DataTypeConversion  OutDataTypeStr=uint8
  VHAL_EPBSta_enum : Outport
  wires:
  UnitConverter/1 -> VHAL_EPBSta_enum/1
  EPBSta/1 -> UnitConverter/1

== system halin/HAL_IN/CAN1/EPS1/DriIntend ==
  DriIntend : Inport
  UnitConverter : DataTypeConversion  OutDataTypeStr=uint8
  VHAL_DriIntend_enum : Outport
  wires:
  UnitConverter/1 -> VHAL_DriIntend_enum/1
  DriIntend/1 -> UnitConverter/1

== system halin/HAL_IN/CAN1/EPS1/EPSAOIControl ==
  EPS_AOI_Control : Inport
  UnitConverter : DataTypeConversion  OutDataTypeStr=uint8
  VHAL_EPSAOIControl_enum : Outport
  wires:
  UnitConverter/1 -> VHAL_EPSAOIControl_enum/1
  EPS_AOI_Control/1 -> UnitConverter/1

== system halin/HAL_IN/CAN1/EPS1/EpasFailed ==
  EpasFailed : Inport
  UnitConverter : DataTypeConversion  OutDataTypeStr=uint8
  VHAL_EpasFailed_enum : Outport
  wires:
  UnitConverter/1 -> VHAL_EpasFailed_enum/1
  EpasFailed/1 -> UnitConverter/1

== system halin/HAL_IN/CAN1/EPS1/SASAngle ==
  SAS_Angle : Inport
  UnitConverter : DataTypeConversion  OutDataTypeStr=uint16
  convert_in : FVT_lib/hal/convert_in  gain=0.1  offset=-900
  VHAL_SASAngle_Deg : Outport
  wires:
  convert_in/1 -> VHAL_SASAngle_Deg/1
  UnitConverter/1 -> convert_in/1
  SAS_Angle/1 -> UnitConverter/1

== system halin/HAL_IN/CAN1/EPS1/SASCAL ==
  SAS_CAL : Inport
  UnitConverter : DataTypeConversion  OutDataTypeStr=uint8
  VHAL_SASCAL_flg : Outport
  wires:
  UnitConverter/1 -> VHAL_SASCAL_flg/1
  SAS_CAL/1 -> UnitConverter/1

== system halin/HAL_IN/CAN1/EPS1/SASSpeed ==
  SAS_Speed : Inport
  UnitConverter : DataTypeConversion  OutDataTypeStr=uint8
  convert_in : FVT_lib/hal/convert_in  gain=4  offset=0
  VHAL_SASSpeed_degps : Outport
  wires:
  convert_in/1 -> VHAL_SASSpeed_degps/1
  UnitConverter/1 -> convert_in/1
  SAS_Speed/1 -> UnitConverter/1

== system halin/HAL_IN/CAN1/EPS1/SASSpeedValid ==
  SAS_Speed_Valid : Inport
  UnitConverter : DataTypeConversion  OutDataTypeStr=uint8
  VHAL_SASSpeedValid_flg : Outport
  wires:
  UnitConverter/1 -> VHAL_SASSpeedValid_flg/1
  SAS_Speed_Valid/1 -> UnitConverter/1

== system halin/HAL_IN/CAN1/EPS1/SASV ==
  SAS_V : Inport
  UnitConverter : DataTypeConversion  OutDataTypeStr=uint8
  VHAL_SASV_flg : Outport
  wires:
  UnitConverter/1 -> VHAL_SASV_flg/1
  SAS_V/1 -> UnitConverter/1

== system halin/HAL_IN/CAN1/ESC1/ABSActive ==
  ABS_Active : Inport
  UnitConverter : DataTypeConversion  OutDataTypeStr=uint8
  VHAL_ABSActive_flg : Outport
  wires:
  UnitConverter/1 -> VHAL_ABSActive_flg/1
  ABS_Active/1 -> UnitConverter/1

== system halin/HAL_IN/CAN1/ESC1/ABSFailed ==
  ABS_Failed : Inport
  UnitConverter : DataTypeConversion  OutDataTypeStr=uint8
  VHAL_ABSFailed_flg : Outport
  wires:
  UnitConverter/1 -> VHAL_ABSFailed_flg/1
  ABS_Failed/1 -> UnitConverter/1

== system halin/HAL_IN/CAN1/ESC1/ABSWnlmpSta ==
  ABS_WnlmpSta : Inport
  UnitConverter : DataTypeConversion  OutDataTypeStr=uint8
  VHAL_ABSWnlmpSta_flg : Outport
  wires:
  UnitConverter/1 -> VHAL_ABSWnlmpSta_flg/1
  ABS_WnlmpSta/1 -> UnitConverter/1

== system halin/HAL_IN/CAN1/ESC1/AVHActive ==
  AVH_Active : Inport
  UnitConverter : DataTypeConversion  OutDataTypeStr=uint8
  VHAL_AVHActive_flg : Outport
  wires:
  UnitConverter/1 -> VHAL_AVHActive_flg/1
  AVH_Active/1 -> UnitConverter/1

== system halin/HAL_IN/CAN1/ESC1/AVHFailed ==
  AVH_Failed : Inport
  UnitConverter : DataTypeConversion  OutDataTypeStr=uint8
  VHAL_AVHFailed_flg : Outport
  wires:
  UnitConverter/1 -> VHAL_AVHFailed_flg/1
  AVH_Failed/1 -> UnitConverter/1

== system halin/HAL_IN/CAN1/ESC1/AmberWnlmpSta ==
  Amber_WnlmpSta : Inport
  UnitConverter : DataTypeConversion  OutDataTypeStr=uint8
  VHAL_AmberWnlmpSta_flg : Outport
  wires:
  UnitConverter/1 -> VHAL_AmberWnlmpSta_flg/1
  Amber_WnlmpSta/1 -> UnitConverter/1

== system halin/HAL_IN/CAN1/ESC1/BTCSActive ==
  BTCS_Active : Inport
  UnitConverter : DataTypeConversion  OutDataTypeStr=uint8
  VHAL_BTCSActive_flg : Outport
  wires:
  UnitConverter/1 -> VHAL_BTCSActive_flg/1
  BTCS_Active/1 -> UnitConverter/1

== system halin/HAL_IN/CAN1/ESC1/EBDActive ==
  EBD_Active : Inport
  UnitConverter : DataTypeConversion  OutDataTypeStr=uint8
  VHAL_EBDActive_flg : Outport
  wires:
  UnitConverter/1 -> VHAL_EBDActive_flg/1
  EBD_Active/1 -> UnitConverter/1

== system halin/HAL_IN/CAN1/ESC1/EBDFailed ==
  EBD_Failed : Inport
  UnitConverter : DataTypeConversion  OutDataTypeStr=uint8
  VHAL_EBDFailed_flg : Outport
  wires:
  UnitConverter/1 -> VHAL_EBDFailed_flg/1
  EBD_Failed/1 -> UnitConverter/1

== system halin/HAL_IN/CAN1/ESC1/ESC1CS ==
  ESC1_CS : Inport
  UnitConverter : DataTypeConversion  OutDataTypeStr=uint8
  VHAL_ESC1CS_enum : Outport
  wires:
  UnitConverter/1 -> VHAL_ESC1CS_enum/1
  ESC1_CS/1 -> UnitConverter/1

== system halin/HAL_IN/CAN1/ESC1/ESC1RC ==
  ESC1_RC : Inport
  UnitConverter : DataTypeConversion  OutDataTypeStr=uint8
  VHAL_ESC1RC_enum : Outport
  wires:
  UnitConverter/1 -> VHAL_ESC1RC_enum/1
  ESC1_RC/1 -> UnitConverter/1

== system halin/HAL_IN/CAN1/ESC1/ESCActive ==
  ESC_Active : Inport
  UnitConverter : DataTypeConversion  OutDataTypeStr=uint8
  VHAL_ESCActive_flg : Outport
  wires:
  UnitConverter/1 -> VHAL_ESCActive_flg/1
  ESC_Active/1 -> UnitConverter/1

== system halin/HAL_IN/CAN1/ESC1/ESCBeepReq ==
  ESC_BeepReq : Inport
  UnitConverter : DataTypeConversion  OutDataTypeStr=uint8
  VHAL_ESCBeepReq_flg : Outport
  wires:
  UnitConverter/1 -> VHAL_ESCBeepReq_flg/1
  ESC_BeepReq/1 -> UnitConverter/1

== system halin/HAL_IN/CAN1/ESC1/ESCFailed ==
  ESC_Failed : Inport
  UnitConverter : DataTypeConversion  OutDataTypeStr=uint8
  VHAL_ESCFailed_flg : Outport
  wires:
  UnitConverter/1 -> VHAL_ESCFailed_flg/1
  ESC_Failed/1 -> UnitConverter/1

== system halin/HAL_IN/CAN1/ESC1/ESCOFFStatus ==
  ESC_OFF_Status : Inport
  UnitConverter : DataTypeConversion  OutDataTypeStr=uint8
  VHAL_ESCOFFStatus_enum : Outport
  wires:
  UnitConverter/1 -> VHAL_ESCOFFStatus_enum/1
  ESC_OFF_Status/1 -> UnitConverter/1

== system halin/HAL_IN/CAN1/ESC1/ESCOfflmpSta ==
  ESC_Off_lmpSta : Inport
  UnitConverter : DataTypeConversion  OutDataTypeStr=uint8
  VHAL_ESCOfflmpSta_flg : Outport
  wires:
  UnitConverter/1 -> VHAL_ESCOfflmpSta_flg/1
  ESC_Off_lmpSta/1 -> UnitConverter/1

== system halin/HAL_IN/CAN1/ESC1/ESCWnlmpSta ==
  ESC_WnlmpSta : Inport
  UnitConverter : DataTypeConversion  OutDataTypeStr=uint8
  VHAL_ESCWnlmpSta_enum : Outport
  wires:
  UnitConverter/1 -> VHAL_ESCWnlmpSta_enum/1
  ESC_WnlmpSta/1 -> UnitConverter/1

== system halin/HAL_IN/CAN1/ESC1/ESSActive ==
  ESS_Active : Inport
  UnitConverter : DataTypeConversion  OutDataTypeStr=uint8
  VHAL_ESSActive_flg : Outport
  wires:
  UnitConverter/1 -> VHAL_ESSActive_flg/1
  ESS_Active/1 -> UnitConverter/1

== system halin/HAL_IN/CAN1/ESC1/FrPTCSActive ==
  Fr_PTCS_Active : Inport
  UnitConverter : DataTypeConversion  OutDataTypeStr=uint8
  VHAL_FrPTCSActive_flg : Outport
  wires:
  UnitConverter/1 -> VHAL_FrPTCSActive_flg/1
  Fr_PTCS_Active/1 -> UnitConverter/1

== system halin/HAL_IN/CAN1/ESC1/FrntAxlTrqReqDrv ==
  FrntAxlTrqReq_Drv : Inport
  UnitConverter : DataTypeConversion  OutDataTypeStr=uint16
  convert_in : FVT_lib/hal/convert_in  gain=0.5  offset=-5300
  VHAL_FrntAxlTrqReqDrv_Nm : Outport
  wires:
  convert_in/1 -> VHAL_FrntAxlTrqReqDrv_Nm/1
  UnitConverter/1 -> convert_in/1
  FrntAxlTrqReq_Drv/1 -> UnitConverter/1

== system halin/HAL_IN/CAN1/ESC1/GRADE ==
  GRADE : Inport
  UnitConverter : DataTypeConversion  OutDataTypeStr=uint8
  convert_in : FVT_lib/hal/convert_in  gain=0.35433  offset=-45
  VHAL_GRADE_Deg : Outport
  wires:
  convert_in/1 -> VHAL_GRADE_Deg/1
  UnitConverter/1 -> convert_in/1
  GRADE/1 -> UnitConverter/1

== system halin/HAL_IN/CAN1/ESC1/HBBActive ==
  HBB_Active : Inport
  UnitConverter : DataTypeConversion  OutDataTypeStr=uint8
  VHAL_HBBActive_flg : Outport
  wires:
  UnitConverter/1 -> VHAL_HBBActive_flg/1
  HBB_Active/1 -> UnitConverter/1

== system halin/HAL_IN/CAN1/ESC1/HBBFailed ==
  HBB_Failed : Inport
  UnitConverter : DataTypeConversion  OutDataTypeStr=uint8
  VHAL_HBBFailed_flg : Outport
  wires:
  UnitConverter/1 -> VHAL_HBBFailed_flg/1
  HBB_Failed/1 -> UnitConverter/1

== system halin/HAL_IN/CAN1/ESC1/HDDActive ==
  HDD_Active : Inport
  UnitConverter : DataTypeConversion  OutDataTypeStr=uint8
  VHAL_HDDActive_flg : Outport
  wires:
  UnitConverter/1 -> VHAL_HDDActive_flg/1
  HDD_Active/1 -> UnitConverter/1

== system halin/HAL_IN/CAN1/ESC1/HDDFailed ==
  HDD_Failed : Inport
  UnitConverter : DataTypeConversion  OutDataTypeStr=uint8
  VHAL_HDDFailed_flg : Outport
  wires:
  UnitConverter/1 -> VHAL_HDDFailed_flg/1
  HDD_Failed/1 -> UnitConverter/1

== system halin/HAL_IN/CAN1/ESC1/HSAActive ==
  HSA_Active : Inport
  UnitConverter : DataTypeConversion  OutDataTypeStr=uint8
  VHAL_HSAActive_flg : Outport
  wires:
  UnitConverter/1 -> VHAL_HSAActive_flg/1
  HSA_Active/1 -> UnitConverter/1

== system halin/HAL_IN/CAN1/ESC1/HSAFailed ==
  HSA_Failed : Inport
  UnitConverter : DataTypeConversion  OutDataTypeStr=uint8
  VHAL_HSAFailed_flg : Outport
  wires:
  UnitConverter/1 -> VHAL_HSAFailed_flg/1
  HSA_Failed/1 -> UnitConverter/1

== system halin/HAL_IN/CAN1/ESC1/LFPulseCount ==
  LF_PulseCount : Inport
  UnitConverter : DataTypeConversion  OutDataTypeStr=uint8
  VHAL_LFPulseCount_enum : Outport
  wires:
  UnitConverter/1 -> VHAL_LFPulseCount_enum/1
  LF_PulseCount/1 -> UnitConverter/1

== system halin/HAL_IN/CAN1/ESC1/LFPulseCountV ==
  LF_PulseCount_V : Inport
  UnitConverter : DataTypeConversion  OutDataTypeStr=uint8
  VHAL_LFPulseCountV_flg : Outport
  wires:
  UnitConverter/1 -> VHAL_LFPulseCountV_flg/1
  LF_PulseCount_V/1 -> UnitConverter/1

== system halin/HAL_IN/CAN1/ESC1/LFRawWhlSpeed ==
  LF_RawWhlSpeed : Inport
  UnitConverter : DataTypeConversion  OutDataTypeStr=uint16
  convert_in : FVT_lib/hal/convert_in  gain=0.0625  offset=0
  VHAL_LFRawWhlSpeed_kph : Outport
  wires:
  convert_in/1 -> VHAL_LFRawWhlSpeed_kph/1
  UnitConverter/1 -> convert_in/1
  LF_RawWhlSpeed/1 -> UnitConverter/1

== system halin/HAL_IN/CAN1/ESC1/LFRawWhlSpeedV ==
  LF_RawWhlSpeed_V : Inport
  UnitConverter : DataTypeConversion  OutDataTypeStr=uint8
  VHAL_LFRawWhlSpeedV_flg : Outport
  wires:
  UnitConverter/1 -> VHAL_LFRawWhlSpeedV_flg/1
  LF_RawWhlSpeed_V/1 -> UnitConverter/1

== system halin/HAL_IN/CAN1/ESC1/LFWhlRotDir ==
  LF_WhlRotDir : Inport
  UnitConverter : DataTypeConversion  OutDataTypeStr=uint8
  VHAL_LFWhlRotDir_enum : Outport
  wires:
  UnitConverter/1 -> VHAL_LFWhlRotDir_enum/1
  LF_WhlRotDir/1 -> UnitConverter/1

== system halin/HAL_IN/CAN1/ESC1/LRPulseCount ==
  LR_PulseCount : Inport
  UnitConverter : DataTypeConversion  OutDataTypeStr=uint8
  VHAL_LRPulseCount_enum : Outport
  wires:
  UnitConverter/1 -> VHAL_LRPulseCount_enum/1
  LR_PulseCount/1 -> UnitConverter/1

== system halin/HAL_IN/CAN1/ESC1/LRPulseCountV ==
  LR_PulseCount_V : Inport
  UnitConverter : DataTypeConversion  OutDataTypeStr=uint8
  VHAL_LRPulseCountV_flg : Outport
  wires:
  UnitConverter/1 -> VHAL_LRPulseCountV_flg/1
  LR_PulseCount_V/1 -> UnitConverter/1

== system halin/HAL_IN/CAN1/ESC1/LRRawWhlSpeed ==
  LR_RawWhlSpeed : Inport
  UnitConverter : DataTypeConversion  OutDataTypeStr=uint16
  convert_in : FVT_lib/hal/convert_in  gain=0.0625  offset=0
  VHAL_LRRawWhlSpeed_kph : Outport
  wires:
  convert_in/1 -> VHAL_LRRawWhlSpeed_kph/1
  UnitConverter/1 -> convert_in/1
  LR_RawWhlSpeed/1 -> UnitConverter/1

== system halin/HAL_IN/CAN1/ESC1/LRRawWhlSpeedV ==
  LR_RawWhlSpeed_V : Inport
  UnitConverter : DataTypeConversion  OutDataTypeStr=uint8
  VHAL_LRRawWhlSpeedV_flg : Outport
  wires:
  UnitConverter/1 -> VHAL_LRRawWhlSpeedV_flg/1
  LR_RawWhlSpeed_V/1 -> UnitConverter/1

== system halin/HAL_IN/CAN1/ESC1/LRWhlRotDir ==
  LR_WhlRotDir : Inport
  UnitConverter : DataTypeConversion  OutDataTypeStr=uint8
  VHAL_LRWhlRotDir_enum : Outport
  wires:
  UnitConverter/1 -> VHAL_LRWhlRotDir_enum/1
  LR_WhlRotDir/1 -> UnitConverter/1

== system halin/HAL_IN/CAN1/ESC1/PBAActive ==
  PBA_Active : Inport
  UnitConverter : DataTypeConversion  OutDataTypeStr=uint8
  VHAL_PBAActive_flg : Outport
  wires:
  UnitConverter/1 -> VHAL_PBAActive_flg/1
  PBA_Active/1 -> UnitConverter/1

== system halin/HAL_IN/CAN1/ESC1/PBAFailed ==
  PBA_Failed : Inport
  UnitConverter : DataTypeConversion  OutDataTypeStr=uint8
  VHAL_PBAFailed_flg : Outport
  wires:
  UnitConverter/1 -> VHAL_PBAFailed_flg/1
  PBA_Failed/1 -> UnitConverter/1
